simulink model "train_model_fessko_1"  (R2021b)
settings: Solver=VariableStepAuto  StartTime=0.0  StopTime=10.0  RelTol=1e-3
model workspace (MAT data in the model file):
  g = 9.8
  l = 1
libraries: simulink_extras x1
settings Model: Creator=petr_  LastModifiedBy=petr_
settings DebuggingCC: UnconnectedInputMsg=none  UnconnectedOutputMsg=none  UnconnectedLineMsg=none
settings ModelReferenceCC: EnableRefExpFcnMdlSchedulingChecks=off
settings RTWCC: GPUComputeCapability=5.0  DLArmComputeVersion=20.02.1

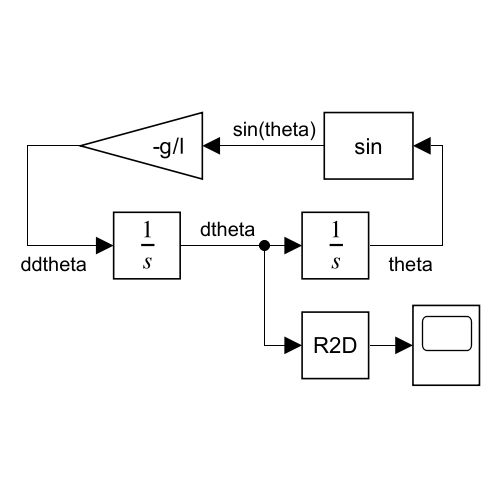
[thumbnail: Simulink's stored preview of the top-level diagram]
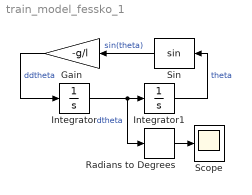
== system train_model_fessko_1 ==
  Gain : Gain  Gain=-g/l
  Integrator : Integrator  InitialCondition=deg2rad(30)
  Integrator1 : Integrator
  Radians to Degrees : simulink_extras/Transformations/Radians to Degrees
  Scope : Scope
  Sin : Trigonometry
  wires:
  Integrator/1 -> Radians to Degrees/1, Integrator1/1  "dtheta"
  Gain/1 -> Integrator/1  "ddtheta"
  Sin/1 -> Gain/1  "sin(theta)"
  Radians to Degrees/1 -> Scope/1
  Integrator1/1 -> Sin/1  "theta"
